simulink model "Tisch"  (R2014b)
settings: Solver=ode45  StartTime=0.0  StopTime=10.0  RelTol=1e-3
settings Model: Creator=Florian  LastModifiedBy=Florian

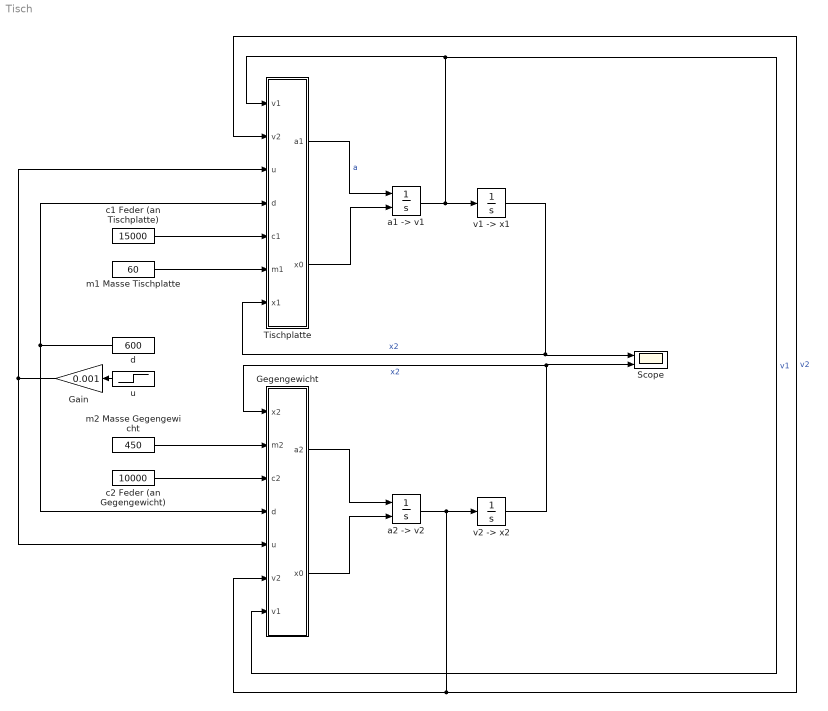
== system Tisch ==
  Gain : Gain  Gain=0.001
  Gegengewicht : MATLAB Function  TreatAsAtomicUnit=on
  "Scope " : Scope  NumInputPorts=2
      settings: YMin=-5~-5  YMax=5~5
  Tischplatte : MATLAB Function  TreatAsAtomicUnit=on
  "a1 -> v1" : Integrator  InitialConditionSource=external
  "a2 -> v2" : Integrator  InitialConditionSource=external
  c1 Feder (an Tischplatte) : Constant  Value=15000
  c2 Feder (an Gegengewicht) : Constant  Value=10000
  d : Constant  Value=600
  m1 Masse Tischplatte : Constant  Value=60
  m2 Masse Gegengewicht : Constant  Value=450
  u : Step  SampleTime=0
  "v1 -> x1" : Integrator
  "v2 -> x2" : Integrator
  wires:
  Tischplatte/1(a1) -> "a1 -> v1"/1  "a"
  "a1 -> v1"/1 -> Gegengewicht/7(v1), Tischplatte/1(v1), "v1 -> x1"/1  "v1"
  Tischplatte/2(x0) -> "a1 -> v1"/2
  "v1 -> x1"/1 -> Tischplatte/7(x1), "Scope "/1  "x2"
  m1 Masse Tischplatte/1 -> Tischplatte/6(m1)
  c1 Feder (an Tischplatte)/1 -> Tischplatte/5(c1)
  d/1 -> Gegengewicht/4(d), Tischplatte/4(d)
  m2 Masse Gegengewicht/1 -> Gegengewicht/2(m2)
  c2 Feder (an Gegengewicht)/1 -> Gegengewicht/3(c2)
  Gegengewicht/1(a2) -> "a2 -> v2"/1
  Gegengewicht/2(x0) -> "a2 -> v2"/2
  "v2 -> x2"/1 -> Gegengewicht/1(x2), "Scope "/2  "x2"
  "a2 -> v2"/1 -> Gegengewicht/6(v2), Tischplatte/2(v2), "v2 -> x2"/1  "v2"
  Gain/1 -> Gegengewicht/5(u), Tischplatte/3(u)
  u/1 -> Gain/1

== matlab function Tisch/Gegengewicht ==
  data: x2 input; m2 input; c2 input; d input; u input; v2 input; v1 input; a2 output; x0 output
function [a2,x0] = fcn(x2,m2,c2,d,u,v2,v1)
g = -9.81; 

Fc = c2*(x2-u);   %Federn
Fd = -d*(v1-v2);  %Dämpfer

a2 = ((m2*g) - (2*Fc) - (2*Fd))/m2; 
x0 = (m2*g)/(2*c2);

== matlab function Tisch/Tischplatte ==
  data: v1 input; v2 input; u input; d input; c1 input; m1 input; x1 input; a1 output; x0 output
function [a1,x0] = fcn(v1, v2, u, d, c1, m1, x1 )
g = -9.81;        

Fc = c1*(x1-u);   %Federn
Fd = -d*(v1-v2);  %Dämpfer

a1 = ((m1*g) - (2*Fc) + (2*Fd))/m1; 
x0 = (m1*g)/(2*c1);
